simulink model "et_robocon_zack_stepup"  (R2013b)
settings: Solver=ode3  SolverMode=SingleTasking  StartTime=0.0  StopTime=inf  RelTol=1e-3
undefined symbols (not defined in the file): balancerStates_Bus0, current_mode_status, current_task_operation_status, DiscIntNeverNeededParam, Init_Bus0, K, lightCalib, R, STATE, TRACK_MODE_LIST, W
libraries: legonxtlib x19, simulink_extras x4, simulink x3, limbo_algorithm_atomic_sub_chart_library x1, line_tracking_algorithm_atomic_sub_chart_library x1, parking_algorithm_atomic_sub_chart_library x1
(part 1 of 2)
settings Model: DataDictionary=marioDict.sldd  ExtModeTrigDuration=2  Creator=mbiesiad  LastModifiedBy=jmodiset
settings ConfigSet: Description=Use this configuration to communicate between two robots. This robot is the master.
settings OptimizationCC: OptimizeModelRefInitCode=on  LifeSpan=1
settings DebuggingCC: UnderspecifiedInitializationDetection=Simplified  SolverPrmCheckMsg=none  ParameterPrecisionLossMsg=none  SignalLabelMismatchMsg=error  NonBusSignalsTreatedAsBus=error
settings HardwareCC: ProdLargestAtomicInteger=Long  ProdLargestAtomicFloat=Float  ProdEndianess=LittleEndian  ProdHWDeviceType=ARM Compatible->ARM 7
settings RTWCC: SystemTargetFile=realtime.tlc  GenerateMakefile=off  TemplateMakefile=realtime.tmf  Description=Run on Target Hardware  RTWVerbose=off  ProcessScript=realtime_make_rtw_hook
settings STFCustomTargetCC: TargetLibSuffix=.a  GenerateSampleERTMain=on  ERTCustomFileBanners=on  SupportNonInlinedSFcns=off  SupportVariableSizeSignals=on  MATLABClassNameForMDSCustomization=Simulink.SoftwareTarget.ERTCustomization  GRTInterface=off  SystemTargetFile=realtime.tlc
settings ERTTargetCC: CodeReplacementLibrary=ANSI_C  GenerateSampleERTMain=on  ParMdlRefBuildCompliant=off  CompOptLevelCompliant=off  ConcurrentExecutionCompliant=off  CombineOutputUpdateFcns=off  ERTFirstTimeCompliant=off  SupportContinuousTime=on  SupportVariableSizeSignals=on  ModelStepFunctionPrototypeControlCompliant=off  CPPClassGenCompliant=off  ExtModeTransport=1  ExtModeMexFile=ext_serial_win32_comm_no_acks_rtt_byteswap  ExtModeMexArgs=0 1 9600  InlinedParameterPlacement=NonHierarchical  ERTSrcFileBannerTemplate=realtime_code_template.cgt  ERTHdrFileBannerTemplate=realtime_code_template.cgt  ERTDataSrcFileTemplate=realtime_code_template.cgt  ERTDataHdrFileTemplate=realtime_code_template.cgt  ERTCustomFileTemplate=realtime_file_process.tlc

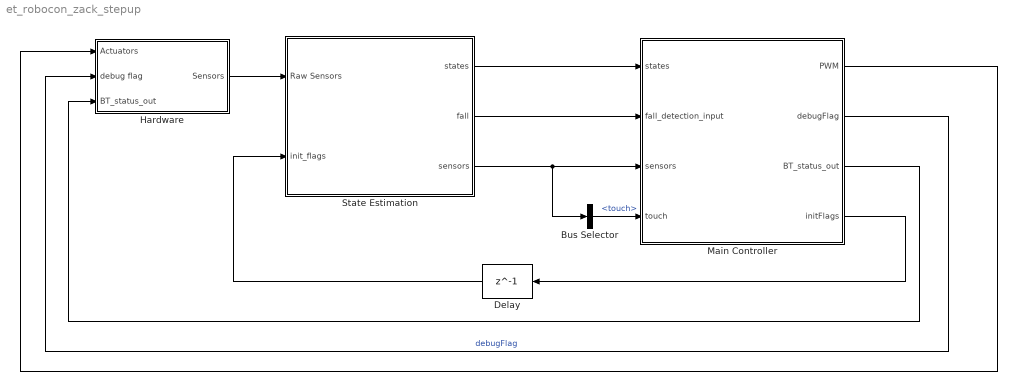
== system et_robocon_zack_stepup ==
  Bus Selector : BusSelector  OutputSignals=touch
  Delay : Delay  DelayLength=1
  Hardware : Subsystem  VariantControl=Variant1
  Main Controller : Stateflow chart  TreatAsAtomicUnit=on
  State Estimation : Subsystem
  wires:
  State Estimation/2(fall) -> Main Controller/2(fall_detection_input)
  State Estimation/3(sensors) -> Bus Selector/1, Main Controller/3(sensors)
  Bus Selector/1 -> Main Controller/4(touch)  "<touch>"
  Hardware/1(Sensors) -> State Estimation/1(Raw Sensors)
  Main Controller/4(initFlags) -> Delay/1
  State Estimation/1(states) -> Main Controller/1(states)
  Delay/1 -> State Estimation/2(init_flags)
  Main Controller/2(debugFlag) -> Hardware/2(debug flag)  "debugFlag"
  Main Controller/1(PWM) -> Hardware/1(Actuators)
  Main Controller/3(BT_status_out) -> Hardware/3(BT_status_out)

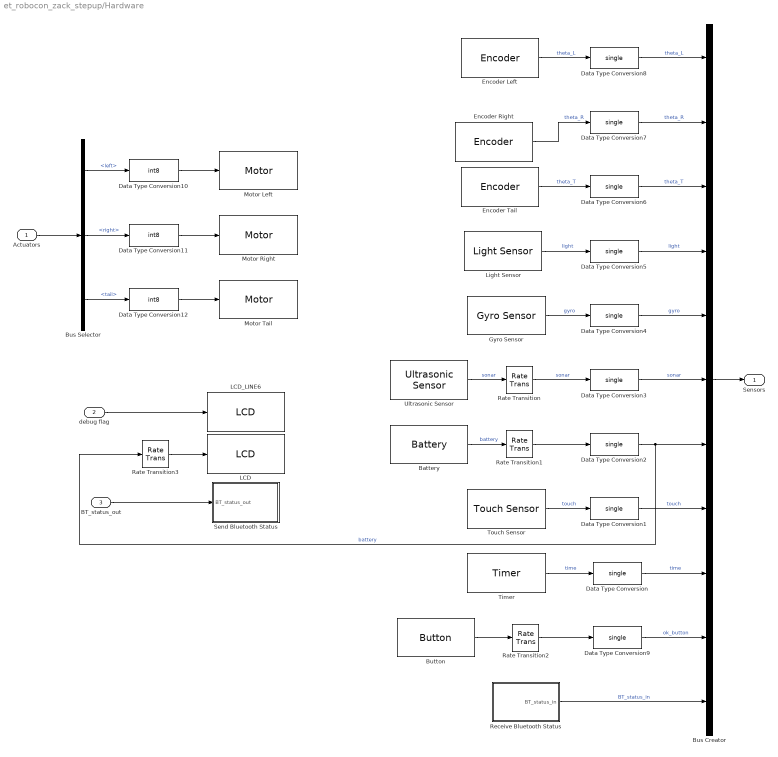
== system et_robocon_zack_stepup/Hardware ==
  Actuators : Inport
  debug flag : Inport  Port=2
  BT_status_out : Inport  Port=3
  Battery : legonxtlib/Battery  sampleTime=.1
  Bus Creator : BusCreator  Inputs=11
  Bus Selector : BusSelector  OutputSignals=left,right,tail
  Button : legonxtlib/Button  buttonType=Middle orange  sampleTime=0.1
  Data Type Conversion{,1..9} (10 alike) : DataTypeConversion  OutDataTypeStr=single
  Data Type Conversion10 : DataTypeConversion  OutDataTypeStr=int8  SaturateOnIntegerOverflow=on
  Data Type Conversion11 : DataTypeConversion  OutDataTypeStr=int8  SaturateOnIntegerOverflow=on
  Data Type Conversion12 : DataTypeConversion  OutDataTypeStr=int8  SaturateOnIntegerOverflow=on
  Encoder Left : legonxtlib/Encoder  portNumber=C  opMode=No reset  sampleTime=0.004
  Encoder Right : legonxtlib/Encoder  portNumber=B  opMode=No reset  sampleTime=0.004
  Encoder Tail : legonxtlib/Encoder  portNumber=A  opMode=No reset  sampleTime=0.004
  Gyro Sensor : legonxtlib/Gyro Sensor  portNumber=1  outputMode=Rotation rate (-360 - 360)  offset=600  sampleTime=0.004
  LCD : legonxtlib/LCD  slcdStr=Battery  slcdLine=2  slcdFormat=Decimal
  LCD_LINE6 : legonxtlib/LCD  slcdStr=STATE:  slcdLine=1  slcdFormat=Decimal
  Light Sensor : legonxtlib/Light Sensor  portNumber=3  outputMode=Raw A/D (1023 - 0)  lightOn=on  sampleTime=0.004
  Motor Left : legonxtlib/Motor  sportNumber=C  sstopAction=Brake
  Motor Right : legonxtlib/Motor  sportNumber=B  sstopAction=Brake
  Motor Tail : legonxtlib/Motor  sportNumber=A  sstopAction=Brake
  Rate Transition : RateTransition  OutPortSampleTime=0.004
  Rate Transition1 : RateTransition  OutPortSampleTime=0.004
  Rate Transition2 : RateTransition  OutPortSampleTime=0.004
  Rate Transition3 : RateTransition  OutPortSampleTime=3
  Receive Bluetooth Status : Subsystem  Variant=on
  Send Bluetooth Status : Subsystem  Variant=on
  Timer : legonxtlib/Timer  sampleTime=0.004
  Touch Sensor : legonxtlib/Touch Sensor  portNumber=4  sampleTime=0.004
  Ultrasonic Sensor : legonxtlib/Ultrasonic Sensor  PortNumber=2  sampleTime=0.02
  Sensors : Outport
  wires:
  Receive Bluetooth Status/1(BT_status_in) -> Bus Creator/11  "BT_status_in"
  debug flag/1 -> LCD_LINE6/1
  Data Type Conversion9/1 -> Bus Creator/10  "ok_button"
  Rate Transition2/1 -> Data Type Conversion9/1
  Button/1 -> Rate Transition2/1
  Rate Transition1/1 -> Data Type Conversion2/1
  Data Type Conversion8/1 -> Bus Creator/1  "theta_L"
  Data Type Conversion7/1 -> Bus Creator/2  "theta_R"
  Data Type Conversion6/1 -> Bus Creator/3  "theta_T"
  Data Type Conversion5/1 -> Bus Creator/4  "light"
  Data Type Conversion4/1 -> Bus Creator/5  "gyro"
  Data Type Conversion3/1 -> Bus Creator/6  "sonar"
  Data Type Conversion2/1 -> Rate Transition3/1, Bus Creator/7  "battery"
  Data Type Conversion1/1 -> Bus Creator/8  "touch"
  Data Type Conversion/1 -> Bus Creator/9  "time"
  Rate Transition/1 -> Data Type Conversion3/1  "sonar"
  Ultrasonic Sensor/1 -> Rate Transition/1  "sonar"
  Bus Selector/3 -> Data Type Conversion12/1  "<tail>"
  Encoder Tail/1 -> Data Type Conversion6/1  "theta_T"
  Light Sensor/1 -> Data Type Conversion5/1  "light"
  Bus Selector/2 -> Data Type Conversion11/1  "<right>"
  Bus Selector/1 -> Data Type Conversion10/1  "<left>"
  Touch Sensor/1 -> Data Type Conversion1/1  "touch"
  Bus Creator/1 -> Sensors/1
  Battery/1 -> Rate Transition1/1  "battery"
  Gyro Sensor/1 -> Data Type Conversion4/1  "gyro"
  Encoder Right/1 -> Data Type Conversion7/1  "theta_R"
  Encoder Left/1 -> Data Type Conversion8/1  "theta_L"
  Timer/1 -> Data Type Conversion/1  "time"
  Actuators/1 -> Bus Selector/1
  Data Type Conversion10/1 -> Motor Left/1
  Data Type Conversion11/1 -> Motor Right/1
  Data Type Conversion12/1 -> Motor Tail/1
  BT_status_out/1 -> Send Bluetooth Status/1(BT_status_out)
  Rate Transition3/1 -> LCD/1

== system et_robocon_zack_stepup/Main Controller/normal_operation_modes.gyro_calibration_mode ==
  sensors : Inport
  touch : Inport  Port=2
  " Demux " : Demux  Outputs=2
  " SFunction " : S-Function  Tag=Stateflow S-Function et_robocon_zack_stepup 5  FunctionName=sf_sfun  PortCounts=[3 6]  EnableBusSupport=off
  gyro_calibration_mode.GyroCalibration.Speak : Subsystem
      settings: UndoDeleteFcn=Stateflow.SLINSF.SimulinkMan.restorePreDeleteFcn  PreDeleteFcn=Stateflow.SLINSF.SimulinkMan.removePreDeleteFcn
  gyro_calibration_mode.GyroCalibration.tail_controller : Subsystem
      settings: UndoDeleteFcn=Stateflow.SLINSF.SimulinkMan.restorePreDeleteFcn  PreDeleteFcn=Stateflow.SLINSF.SimulinkMan.removePreDeleteFcn
  debugFlag : Outport
  initFlags : Outport  Port=2
  PWM : Outport  Port=3
  wires:
  sensors/1 -> " SFunction "/1
  touch/1 -> " SFunction "/2
  " SFunction "/2 -> debugFlag/1  "debugFlag"
  " SFunction "/3 -> initFlags/1  "initFlags"
  " SFunction "/4 -> PWM/1  "PWM"
  " SFunction "/5 -> gyro_calibration_mode.GyroCalibration.tail_controller/1(current)
  " SFunction "/6 -> gyro_calibration_mode.GyroCalibration.tail_controller/2(desired)
  gyro_calibration_mode.GyroCalibration.tail_controller/1(cmd) -> " SFunction "/3
  " Demux "/1 -> gyro_calibration_mode.GyroCalibration.tail_controller/Trigger
  " Demux "/2 -> gyro_calibration_mode.GyroCalibration.Speak/Trigger
  " SFunction "/1 -> " Demux "/1

== system et_robocon_zack_stepup/Main Controller/normal_operation_modes.light_sensor_calibration_mode ==
  sensors : Inport
  touch : Inport  Port=2
  " Demux " : Demux  Outputs=1
  " SFunction " : S-Function  Tag=Stateflow S-Function et_robocon_zack_stepup 6  FunctionName=sf_sfun  PortCounts=[3 5]  EnableBusSupport=off
  light_sensor_calibration_mode.tail_controller : Subsystem
      settings: UndoDeleteFcn=Stateflow.SLINSF.SimulinkMan.restorePreDeleteFcn  PreDeleteFcn=Stateflow.SLINSF.SimulinkMan.removePreDeleteFcn
  debugFlag : Outport
  PWM : Outport  Port=2
  wires:
  sensors/1 -> " SFunction "/1
  touch/1 -> " SFunction "/2
  " SFunction "/2 -> debugFlag/1  "debugFlag"
  " SFunction "/3 -> PWM/1  "PWM"
  " SFunction "/4 -> light_sensor_calibration_mode.tail_controller/1(current)
  " SFunction "/5 -> light_sensor_calibration_mode.tail_controller/2(desired)
  light_sensor_calibration_mode.tail_controller/1(cmd) -> " SFunction "/3
  " Demux "/1 -> light_sensor_calibration_mode.tail_controller/Trigger
  " SFunction "/1 -> " Demux "/1

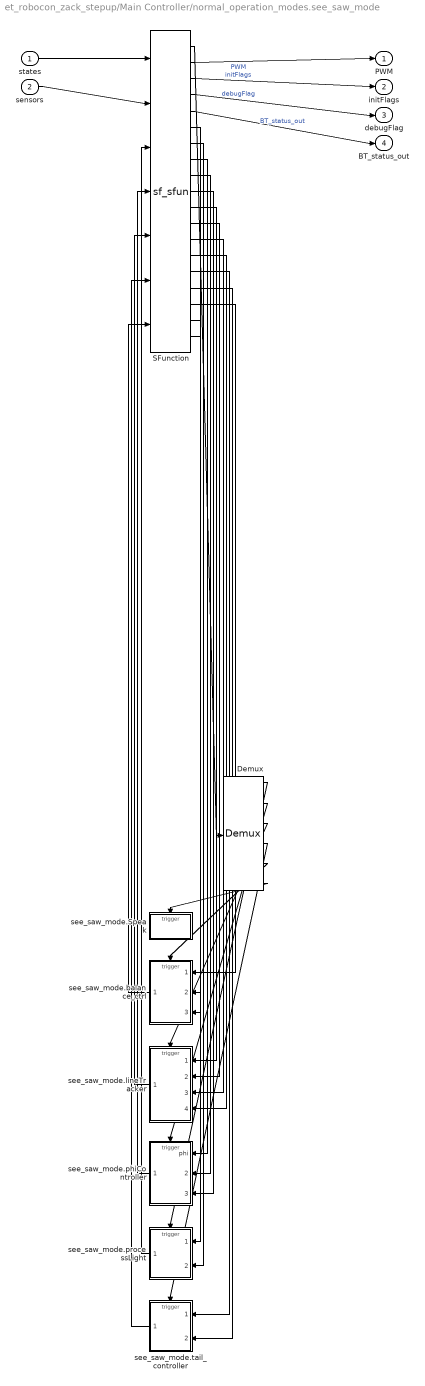
== system et_robocon_zack_stepup/Main Controller/normal_operation_modes.see_saw_mode ==
  states : Inport
  sensors : Inport  Port=2
  " Demux " : Demux  Outputs=6
  " SFunction " : S-Function  Tag=Stateflow S-Function et_robocon_zack_stepup 4  FunctionName=sf_sfun  Parameters=balancerStates_Bus0  PortCounts=[7 19]  EnableBusSupport=off
  see_saw_mode.Speak : Subsystem
      settings: UndoDeleteFcn=Stateflow.SLINSF.SimulinkMan.restorePreDeleteFcn  PreDeleteFcn=Stateflow.SLINSF.SimulinkMan.removePreDeleteFcn
  see_saw_mode.balance_ctrl : Subsystem
      settings: UndoDeleteFcn=Stateflow.SLINSF.SimulinkMan.restorePreDeleteFcn  PreDeleteFcn=Stateflow.SLINSF.SimulinkMan.removePreDeleteFcn
  see_saw_mode.lineTracker : Subsystem
      settings: UndoDeleteFcn=Stateflow.SLINSF.SimulinkMan.restorePreDeleteFcn  PreDeleteFcn=Stateflow.SLINSF.SimulinkMan.removePreDeleteFcn
  see_saw_mode.phiController : Subsystem
      settings: UndoDeleteFcn=Stateflow.SLINSF.SimulinkMan.restorePreDeleteFcn  PreDeleteFcn=Stateflow.SLINSF.SimulinkMan.removePreDeleteFcn
  see_saw_mode.processLight : Subsystem
      settings: UndoDeleteFcn=Stateflow.SLINSF.SimulinkMan.restorePreDeleteFcn  PreDeleteFcn=Stateflow.SLINSF.SimulinkMan.removePreDeleteFcn
  see_saw_mode.tail_controller : Subsystem
      settings: UndoDeleteFcn=Stateflow.SLINSF.SimulinkMan.restorePreDeleteFcn  PreDeleteFcn=Stateflow.SLINSF.SimulinkMan.removePreDeleteFcn
  PWM : Outport
  initFlags : Outport  Port=2
  debugFlag : Outport  Port=3
  BT_status_out : Outport  Port=4
  wires:
  states/1 -> " SFunction "/1
  sensors/1 -> " SFunction "/2
  " SFunction "/2 -> PWM/1  "PWM"
  " SFunction "/3 -> initFlags/1  "initFlags"
  " SFunction "/4 -> debugFlag/1  "debugFlag"
  " SFunction "/5 -> BT_status_out/1  "BT_status_out"
  " SFunction "/6 -> see_saw_mode.processLight/1(rawLight)
  " SFunction "/7 -> see_saw_mode.processLight/2(lightCalib)
  see_saw_mode.processLight/1(light) -> " SFunction "/3
  " Demux "/1 -> see_saw_mode.processLight/Trigger
  " SFunction "/8 -> see_saw_mode.phiController/1(phi)
  " SFunction "/9 -> see_saw_mode.phiController/2(desiredPhi)
  " SFunction "/10 -> see_saw_mode.phiController/3(battery)
  see_saw_mode.phiController/1(cmd) -> " SFunction "/4
  " Demux "/2 -> see_saw_mode.phiController/Trigger
  " SFunction "/11 -> see_saw_mode.lineTracker/1(desiredLight)
  " SFunction "/12 -> see_saw_mode.lineTracker/2(light)
  " SFunction "/13 -> see_saw_mode.lineTracker/3(trackingPower)
  " SFunction "/14 -> see_saw_mode.lineTracker/4(battery)
  see_saw_mode.lineTracker/1(cmd) -> " SFunction "/5
  " Demux "/3 -> see_saw_mode.lineTracker/Trigger
  " SFunction "/15 -> see_saw_mode.tail_controller/1(current)
  " SFunction "/16 -> see_saw_mode.tail_controller/2(desired)
  see_saw_mode.tail_controller/1(cmd) -> " SFunction "/6
  " Demux "/4 -> see_saw_mode.tail_controller/Trigger
  " SFunction "/17 -> see_saw_mode.balance_ctrl/1(balancerStates)
  " SFunction "/18 -> see_saw_mode.balance_ctrl/2(desired_velocity)
  " SFunction "/19 -> see_saw_mode.balance_ctrl/3(battery)
  see_saw_mode.balance_ctrl/1(cmd) -> " SFunction "/7
  " Demux "/5 -> see_saw_mode.balance_ctrl/Trigger
  " Demux "/6 -> see_saw_mode.Speak/Trigger
  " SFunction "/1 -> " Demux "/1

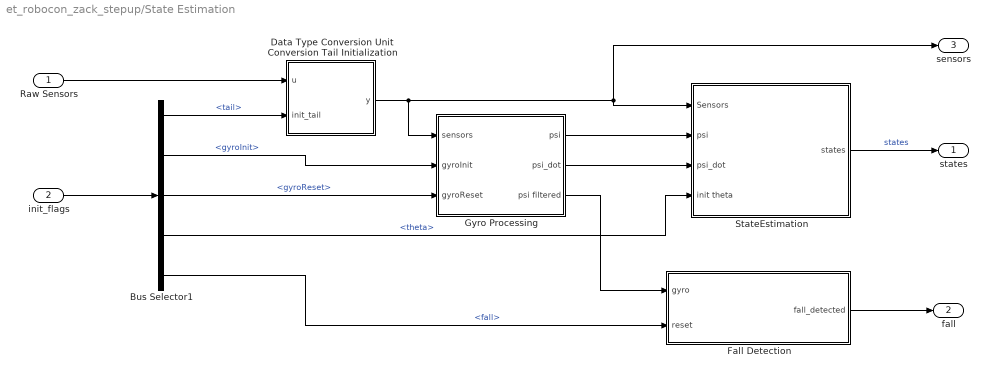
== system et_robocon_zack_stepup/State Estimation ==
  Raw Sensors : Inport
  init_flags : Inport  Port=2
  Bus Selector1 : BusSelector  OutputSignals=tail,gyroInit,gyroReset,theta,fall
  Data Type Conversion Unit Conversion Tail Initialization : Subsystem
  Fall Detection : Subsystem
  Gyro Processing : Subsystem
  StateEstimation : Subsystem
  states : Outport
  fall : Outport  Port=2
  sensors : Outport  Port=3
  wires:
  Bus Selector1/3 -> Gyro Processing/3(gyroReset)  "<gyroReset>"
  Bus Selector1/4 -> StateEstimation/4(init theta)  "<theta>"
  Bus Selector1/1 -> Data Type Conversion Unit Conversion Tail Initialization/2(init_tail)  "<tail>"
  Bus Selector1/2 -> Gyro Processing/2(gyroInit)  "<gyroInit>"
  init_flags/1 -> Bus Selector1/1
  StateEstimation/1(states) -> states/1  "states"
  Data Type Conversion Unit Conversion Tail Initialization/1(y) -> StateEstimation/1(Sensors), sensors/1, Gyro Processing/1(sensors)
  Raw Sensors/1 -> Data Type Conversion Unit Conversion Tail Initialization/1(u)
  Gyro Processing/1(psi) -> StateEstimation/2(psi)
  Gyro Processing/2(psi_dot) -> StateEstimation/3(psi_dot)
  Gyro Processing/3(psi filtered) -> Fall Detection/1(gyro)
  Bus Selector1/5 -> Fall Detection/2(reset)  "<fall>"
  Fall Detection/1(fall_detected) -> fall/1

== system et_robocon_zack_stepup/Hardware/Receive Bluetooth Status ==
  note: 1) Only subsystems can be added as variant choices at this level
      | 2) Blocks cannot be connected at this level as connectivity is
      | automatically determined at simulation, based on the active variant
  BluetoothOFF : Subsystem  VariantControl=BluetoothOFF
  BluetoothON : Subsystem  VariantControl=BluetoothON
  BT_status_in : Outport

== system et_robocon_zack_stepup/Hardware/Send Bluetooth Status ==
  note: 1) Only subsystems can be added as variant choices at this level
      | 2) Blocks cannot be connected at this level as connectivity is
      | automatically determined at simulation, based on the active variant
  BT_status_out : Inport
  BluetoothOFF : Subsystem  VariantControl=BluetoothOFF
  BluetoothON : Subsystem  VariantControl=BluetoothON

== system et_robocon_zack_stepup/Main Controller/normal_operation_modes.gyro_calibration_mode/gyro_calibration_mode.GyroCalibration.Speak ==
  f : TriggerPort  TriggerType=function-call
      settings: CopyFcn=Stateflow.SLINSF.SimulinkMan.removeBlockPreDeleteFcn  PreDeleteFcn=Stateflow.SLINSF.SimulinkMan.unsafePredeleteFcn
  Constant : Constant  Value=50
  Speaker : legonxtlib/Speaker  sinputMode=Volume only  sspeakerFreq=800  sspeakerVolume=50  sspeakerDuration=100
  wires:
  Constant/1 -> Speaker/1

== system et_robocon_zack_stepup/Main Controller/normal_operation_modes.gyro_calibration_mode/gyro_calibration_mode.GyroCalibration.tail_controller ==
  note: Could be improved, PI for example
  current : Inport  OutDataTypeStr=single  PortDimensions=1
  desired : Inport  Port=2  OutDataTypeStr=single  PortDimensions=1
  f : TriggerPort  TriggerType=function-call
      settings: CopyFcn=Stateflow.SLINSF.SimulinkMan.removeBlockPreDeleteFcn  PreDeleteFcn=Stateflow.SLINSF.SimulinkMan.unsafePredeleteFcn
  Gain : Gain  Gain=250
  Saturation : Saturate  UpperLimit=100  LowerLimit=-100  OutDataTypeStr=single
  Sum : Sum  Inputs=|+-
  cmd : Outport  OutDataTypeStr=single  PortDimensions=1  InitialOutput=0
  wires:
  Saturation/1 -> cmd/1
  Gain/1 -> Saturation/1
  desired/1 -> Sum/1
  current/1 -> Sum/2
  Sum/1 -> Gain/1

== system et_robocon_zack_stepup/Main Controller/normal_operation_modes.light_sensor_calibration_mode/light_sensor_calibration_mode.tail_controller ==
  note: Could be improved, PI for example
  current : Inport  OutDataTypeStr=single  PortDimensions=1
  desired : Inport  Port=2  OutDataTypeStr=single  PortDimensions=1
  f : TriggerPort  TriggerType=function-call
      settings: CopyFcn=Stateflow.SLINSF.SimulinkMan.removeBlockPreDeleteFcn  PreDeleteFcn=Stateflow.SLINSF.SimulinkMan.unsafePredeleteFcn
  Gain : Gain  Gain=250
  Saturation : Saturate  UpperLimit=100  LowerLimit=-100  OutDataTypeStr=single
  Sum : Sum  Inputs=|+-
  cmd : Outport  OutDataTypeStr=single  PortDimensions=1  InitialOutput=0
  wires:
  Saturation/1 -> cmd/1
  Gain/1 -> Saturation/1
  desired/1 -> Sum/1
  current/1 -> Sum/2
  Sum/1 -> Gain/1

== system et_robocon_zack_stepup/Main Controller/normal_operation_modes.see_saw_mode/see_saw_mode.Speak ==
  f : TriggerPort  TriggerType=function-call
      settings: CopyFcn=Stateflow.SLINSF.SimulinkMan.removeBlockPreDeleteFcn  PreDeleteFcn=Stateflow.SLINSF.SimulinkMan.unsafePredeleteFcn
  Constant : Constant  Value=50
  Speaker : legonxtlib/Speaker  sinputMode=Volume only  sspeakerFreq=800  sspeakerVolume=50  sspeakerDuration=100
  wires:
  Constant/1 -> Speaker/1

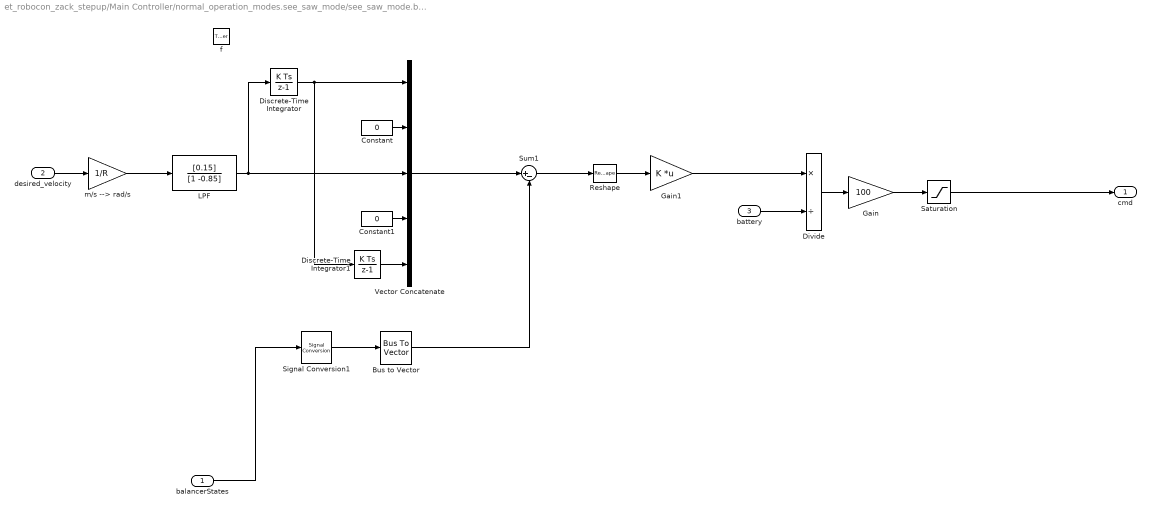
== system et_robocon_zack_stepup/Main Controller/normal_operation_modes.see_saw_mode/see_saw_mode.balance_ctrl ==
  balancerStates : Inport  OutDataTypeStr=Bus: Balancer_States_Bus  PortDimensions=1
  desired_velocity : Inport  Port=2  OutDataTypeStr=single  PortDimensions=1  BusOutputAsStruct=on
  battery : Inport  Port=3  OutDataTypeStr=double  PortDimensions=1
  f : TriggerPort  TriggerType=function-call
      settings: CopyFcn=Stateflow.SLINSF.SimulinkMan.removeBlockPreDeleteFcn  PreDeleteFcn=Stateflow.SLINSF.SimulinkMan.unsafePredeleteFcn
  Bus to Vector : BusToVector
  Constant : Constant  Value=0  OutDataTypeStr=single
  Constant1 : Constant  Value=0  OutDataTypeStr=single
  Discrete-Time Integrator : DiscreteIntegrator  SampleTime=-1  ICPrevOutput=DiscIntNeverNeededParam  ICPrevScaledInput=DiscIntNeverNeededParam
  Discrete-Time Integrator1 : DiscreteIntegrator  SampleTime=-1  ICPrevOutput=DiscIntNeverNeededParam  ICPrevScaledInput=DiscIntNeverNeededParam
  Divide : Product  Inputs=*/
  Gain : Gain  Gain=100
  Gain1 : Gain  Gain=K  Multiplication=Matrix(K*u)
  LPF : DiscreteFilter  Numerator=[0.15]  Denominator=[1 -0.85]
  Reshape : Reshape  OutputDimensionality=Column vector (2-D)
  Saturation : Saturate  UpperLimit=100  LowerLimit=-100  OutDataTypeStr=single
  Signal Conversion1 : SignalConversion  ConversionOutput=Virtual bus
  Sum1 : Sum  Inputs=|+-
  Vector Concatenate : Concatenate  NumInputs=5
  m/s --> rad/s : Gain  Gain=1/R
  cmd : Outport  OutDataTypeStr=single  PortDimensions=1  InitialOutput=0
  wires:
  Discrete-Time Integrator1/1 -> Vector Concatenate/5
  Discrete-Time Integrator/1 -> Vector Concatenate/1, Discrete-Time Integrator1/1
  Constant1/1 -> Vector Concatenate/4
  LPF/1 -> Vector Concatenate/3, Discrete-Time Integrator/1
  Constant/1 -> Vector Concatenate/2
  m/s --> rad/s/1 -> LPF/1
  Signal Conversion1/1 -> Bus to Vector/1
  Divide/1 -> Gain/1
  Gain/1 -> Saturation/1
  Gain1/1 -> Divide/1
  Saturation/1 -> cmd/1
  battery/1 -> Divide/2
  Vector Concatenate/1 -> Sum1/1
  balancerStates/1 -> Signal Conversion1/1
  Bus to Vector/1 -> Sum1/2
  desired_velocity/1 -> m/s --> rad/s/1
  Sum1/1 -> Reshape/1
  Reshape/1 -> Gain1/1

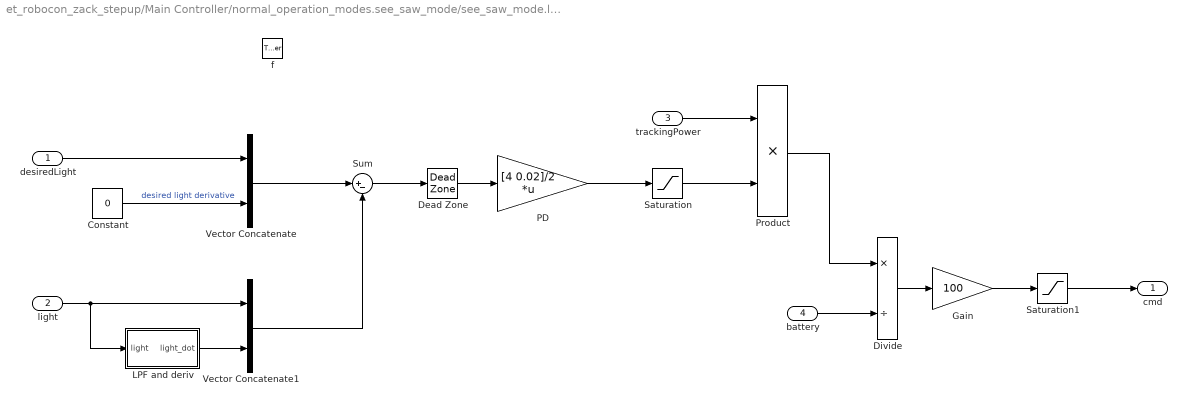
== system et_robocon_zack_stepup/Main Controller/normal_operation_modes.see_saw_mode/see_saw_mode.lineTracker ==
  desiredLight : Inport  OutDataTypeStr=single  PortDimensions=1
  light : Inport  Port=2  OutDataTypeStr=single  PortDimensions=1
  trackingPower : Inport  Port=3  OutDataTypeStr=single  PortDimensions=1
  battery : Inport  Port=4  OutDataTypeStr=double  PortDimensions=1
  f : TriggerPort  TriggerType=function-call
      settings: CopyFcn=Stateflow.SLINSF.SimulinkMan.removeBlockPreDeleteFcn  PreDeleteFcn=Stateflow.SLINSF.SimulinkMan.unsafePredeleteFcn
  Constant : Constant  Value=0  OutDataTypeStr=single
  Dead Zone : DeadZone  LowerValue=-0.02  UpperValue=0.02  SaturateOnIntegerOverflow=on
  Divide : Product  Inputs=*/
  Gain : Gain  Gain=100
  LPF and deriv : Subsystem
  PD : Gain  Gain="[4  0.02]/2"  Multiplication=Matrix(K*u)
  Product : Product
  Saturation : Saturate  UpperLimit=6  LowerLimit=-6
  Saturation1 : Saturate  UpperLimit=100  LowerLimit=-100  OutDataTypeStr=single
  Sum : Sum  Inputs=|+-
  Vector Concatenate : Concatenate
  Vector Concatenate1 : Concatenate
  cmd : Outport  OutDataTypeStr=single  PortDimensions=1
  wires:
  Divide/1 -> Gain/1
  Gain/1 -> Saturation1/1
  battery/1 -> Divide/2
  Saturation1/1 -> cmd/1
  Product/1 -> Divide/1
  trackingPower/1 -> Product/1
  Saturation/1 -> Product/2
  PD/1 -> Saturation/1
  Dead Zone/1 -> PD/1
  Sum/1 -> Dead Zone/1
  Vector Concatenate1/1 -> Sum/2
  Vector Concatenate/1 -> Sum/1
  light/1 -> Vector Concatenate1/1, LPF and deriv/1(light)
  LPF and deriv/1(light_dot) -> Vector Concatenate1/2
  Constant/1 -> Vector Concatenate/2  "desired light derivative"
  desiredLight/1 -> Vector Concatenate/1

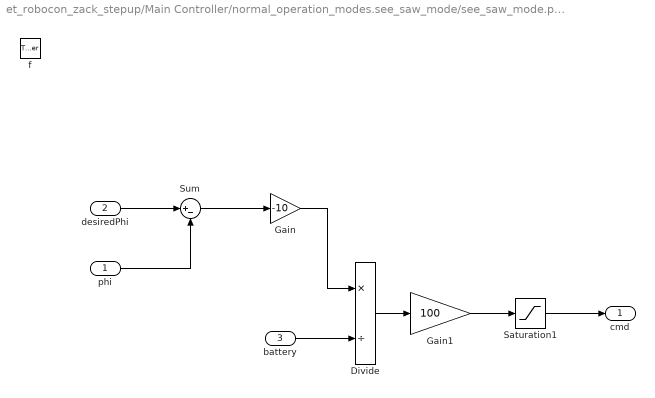
== system et_robocon_zack_stepup/Main Controller/normal_operation_modes.see_saw_mode/see_saw_mode.phiController ==
  phi : Inport  OutDataTypeStr=single  PortDimensions=1
  desiredPhi : Inport  Port=2  OutDataTypeStr=single  PortDimensions=1
  battery : Inport  Port=3  OutDataTypeStr=double  PortDimensions=1
  f : TriggerPort  TriggerType=function-call
      settings: CopyFcn=Stateflow.SLINSF.SimulinkMan.removeBlockPreDeleteFcn  PreDeleteFcn=Stateflow.SLINSF.SimulinkMan.unsafePredeleteFcn
  Divide : Product  Inputs=*/
  Gain : Gain  Gain=-10
  Gain1 : Gain  Gain=100
  Saturation1 : Saturate  UpperLimit=100  LowerLimit=-100  OutDataTypeStr=single
  Sum : Sum  Inputs=|+-
  cmd : Outport
  wires:
  Saturation1/1 -> cmd/1
  Gain/1 -> Divide/1
  Divide/1 -> Gain1/1
  Gain1/1 -> Saturation1/1
  battery/1 -> Divide/2
  Sum/1 -> Gain/1
  phi/1 -> Sum/2
  desiredPhi/1 -> Sum/1

== system et_robocon_zack_stepup/Main Controller/normal_operation_modes.see_saw_mode/see_saw_mode.processLight ==
  rawLight : Inport  OutDataTypeStr=single  PortDimensions=1
  lightCalib : Inport  Port=2  OutDataTypeStr=Bus: Light_Bus  PortDimensions=1
  f : TriggerPort  TriggerType=function-call
      settings: CopyFcn=Stateflow.SLINSF.SimulinkMan.removeBlockPreDeleteFcn  PreDeleteFcn=Stateflow.SLINSF.SimulinkMan.unsafePredeleteFcn
  Bus Selector : BusSelector  OutputSignals=black,white
  Gain : Gain  Gain=0.3
  Gain1 : Gain  Gain=1/100
  Sum : Sum  Inputs=|+-
  Sum1 : Sum  Inputs=|++
  Sum2 : Sum  Inputs=|+-
  light : Outport
  wires:
  Gain1/1 -> light/1
  Sum2/1 -> Gain1/1
  Sum1/1 -> Sum2/2
  rawLight/1 -> Sum2/1
  Gain/1 -> Sum1/1
  Sum/1 -> Gain/1
  Bus Selector/2 -> Sum/2, Sum1/2  "<white>"
  Bus Selector/1 -> Sum/1  "<black>"
  lightCalib/1 -> Bus Selector/1

== system et_robocon_zack_stepup/Main Controller/normal_operation_modes.see_saw_mode/see_saw_mode.tail_controller ==
  note: Could be improved, PI for example
  current : Inport  OutDataTypeStr=single  PortDimensions=1
  desired : Inport  Port=2  OutDataTypeStr=single  PortDimensions=1
  f : TriggerPort  TriggerType=function-call
      settings: CopyFcn=Stateflow.SLINSF.SimulinkMan.removeBlockPreDeleteFcn  PreDeleteFcn=Stateflow.SLINSF.SimulinkMan.unsafePredeleteFcn
  Gain : Gain  Gain=250
  Saturation : Saturate  UpperLimit=100  LowerLimit=-100  OutDataTypeStr=single
  Sum : Sum  Inputs=|+-
  cmd : Outport  OutDataTypeStr=single  PortDimensions=1  InitialOutput=0
  wires:
  Saturation/1 -> cmd/1
  Gain/1 -> Saturation/1
  desired/1 -> Sum/1
  current/1 -> Sum/2
  Sum/1 -> Gain/1

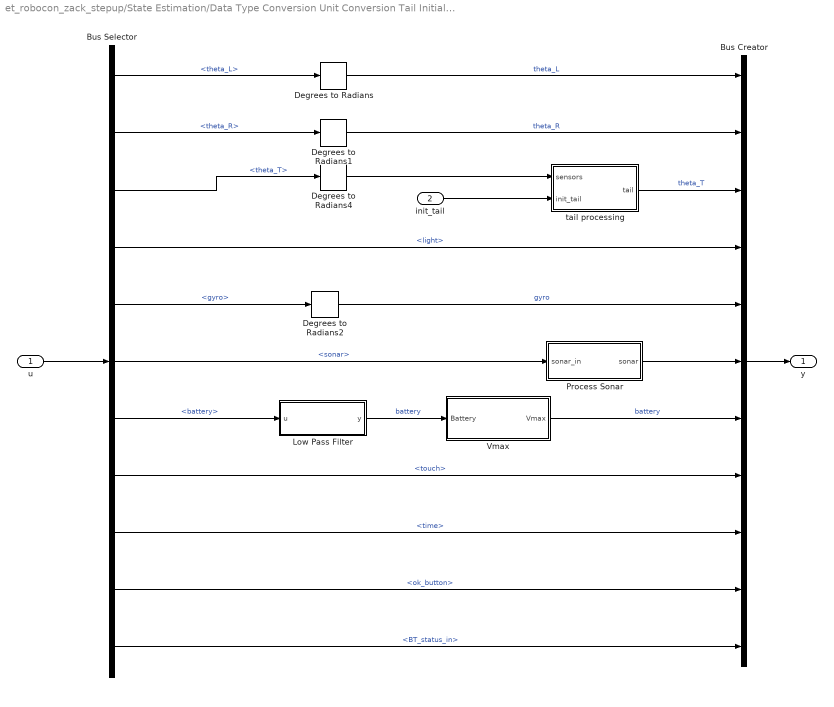
== system et_robocon_zack_stepup/State Estimation/Data Type Conversion Unit Conversion Tail Initialization ==
  u : Inport
  init_tail : Inport  Port=2
  Bus Creator : BusCreator  Inputs=11  OutDataTypeStr=Bus: Sensors_Bus
  Bus Selector : BusSelector  OutputSignals=theta_L,theta_R,theta_T,light,gyro,sonar,battery,touch,time,ok_button,BT_status_in
  Degrees to Radians{,1..2,4} (4 alike) : simulink_extras/Transformations/Degrees to Radians
  Low Pass Filter : Subsystem
  Process Sonar : Subsystem
  Vmax : Subsystem
  tail processing : Subsystem
  y : Outport
  wires:
  Bus Selector/11 -> Bus Creator/11  "<BT_status_in>"
  Process Sonar/1(sonar) -> Bus Creator/6
  Bus Selector/6 -> Process Sonar/1(sonar_in)  "<sonar>"
  Bus Selector/10 -> Bus Creator/10  "<ok_button>"
  init_tail/1 -> tail processing/2(init_tail)
  Bus Selector/9 -> Bus Creator/9  "<time>"
  Bus Selector/8 -> Bus Creator/8  "<touch>"
  tail processing/1(tail) -> Bus Creator/3  "theta_T"
  Degrees to Radians4/1 -> tail processing/1(sensors)
  Vmax/1(Vmax) -> Bus Creator/7  "battery"
  Degrees to Radians2/1 -> Bus Creator/5  "gyro"
  Bus Selector/3 -> Degrees to Radians4/1  "<theta_T>"
  Bus Selector/7 -> Low Pass Filter/1(u)  "<battery>"
  Bus Selector/5 -> Degrees to Radians2/1  "<gyro>"
  Bus Selector/4 -> Bus Creator/4  "<light>"
  Bus Creator/1 -> y/1
  u/1 -> Bus Selector/1
  Degrees to Radians/1 -> Bus Creator/1  "theta_L"
  Bus Selector/2 -> Degrees to Radians1/1  "<theta_R>"
  Bus Selector/1 -> Degrees to Radians/1  "<theta_L>"
  Low Pass Filter/1(y) -> Vmax/1(Battery)  "battery"
  Degrees to Radians1/1 -> Bus Creator/2  "theta_R"

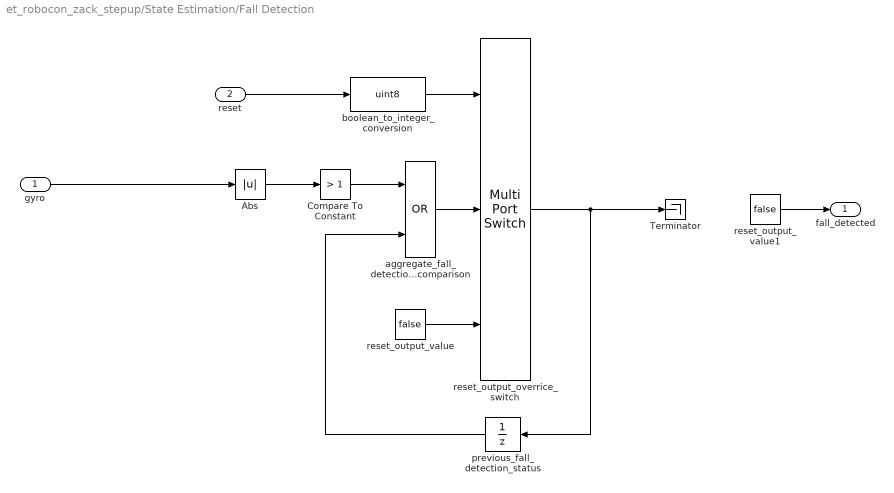
== system et_robocon_zack_stepup/State Estimation/Fall Detection ==
  gyro : Inport
      settings: AttributesFormatString=Output data type: %<OutDataTypeStr>
  reset : Inport  Port=2  OutDataTypeStr=boolean
      settings: AttributesFormatString=Output data type: %<OutDataTypeStr>
  Abs : Abs
  Compare To Constant : simulink/Logic and Bit Operations/Compare To Constant  relop=>  const=1  OutDataTypeStr=boolean
  Terminator : Terminator
  aggregate_fall_detection_comparison : Logic  Operator=OR  OutDataTypeStr=boolean
  boolean_to_integer_conversion : DataTypeConversion  OutDataTypeStr=uint8
      settings: AttributesFormatString=Output data type: %<OutDataTypeStr>
  previous_fall_detection_status : UnitDelay  SampleTime=-1
  reset_output_overrice_switch : MultiPortSwitch  DataPortOrder=Zero-based contiguous  Inputs=2  zeroidx=on  InputSameDT=on
  reset_output_value : Constant  Value=false
  reset_output_value1 : Constant  Value=false
  fall_detected : Outport
  wires:
  reset_output_overrice_switch/1 -> Terminator/1, previous_fall_detection_status/1
  reset_output_value/1 -> reset_output_overrice_switch/3
  aggregate_fall_detection_comparison/1 -> reset_output_overrice_switch/2
  boolean_to_integer_conversion/1 -> reset_output_overrice_switch/1
  reset/1 -> boolean_to_integer_conversion/1
  previous_fall_detection_status/1 -> aggregate_fall_detection_comparison/2
  Abs/1 -> Compare To Constant/1
  gyro/1 -> Abs/1
  Compare To Constant/1 -> aggregate_fall_detection_comparison/1
  reset_output_value1/1 -> fall_detected/1

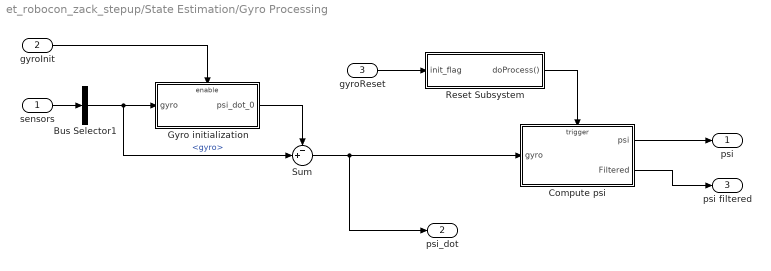
== system et_robocon_zack_stepup/State Estimation/Gyro Processing ==
  sensors : Inport
  gyroInit : Inport  Port=2
  gyroReset : Inport  Port=3
  Bus Selector1 : BusSelector  OutputSignals=gyro
  Compute psi : Subsystem
  Gyro initialization : Subsystem  TreatAsAtomicUnit=on
  Reset Subsystem : Stateflow chart  TreatAsAtomicUnit=on
  Sum : Sum  Inputs=-+|
  psi : Outport
  psi_dot : Outport  Port=2
  psi filtered : Outport  Port=3
  wires:
  Compute psi/2(Filtered) -> psi filtered/1
  Reset Subsystem/1(doProcess()) -> Compute psi/Trigger
  gyroReset/1 -> Reset Subsystem/1(init_flag)
  Bus Selector1/1 -> Sum/2, Gyro initialization/1(gyro)  "<gyro>"
  Gyro initialization/1(psi_dot_0) -> Sum/1
  Sum/1 -> psi_dot/1, Compute psi/1(gyro)
  Compute psi/1(psi) -> psi/1
  sensors/1 -> Bus Selector1/1
  gyroInit/1 -> Gyro initialization/Enable

== system et_robocon_zack_stepup/State Estimation/StateEstimation ==
  note: Conversion from Raw Sensors to States as described in "NXTway plant model.pdf"
  Sensors : Inport
  psi : Inport  Port=2
  psi_dot : Inport  Port=3
  init theta : Inport  Port=4
  Bus Creator1 : BusCreator  OutDataTypeStr=Bus: States_Bus
  Bus Creator2 : BusCreator  Inputs=5  OutDataTypeStr=Bus: Balancer_States_Bus
  Bus Selector1 : BusSelector  OutputSignals=theta_L,theta_R
  Process theta1 : Subsystem
  Reset Subsystem : Stateflow chart  TreatAsAtomicUnit=on
  states : Outport  OutputWhenDisabled=reset  InitialOutput=0
  wires:
  Process theta1/2(psi_out) -> Bus Creator2/2  "psi"
  Reset Subsystem/1(doProcess()) -> Process theta1/Trigger
  Bus Selector1/2 -> Process theta1/3(theta_r)  "<theta_R>"
  Bus Selector1/1 -> Process theta1/2(theta_l)  "<theta_L>"
  init theta/1 -> Reset Subsystem/1(init_flag)
  Process theta1/1(theta) -> Bus Creator2/1  "theta"
  Process theta1/3(theta_dot) -> Bus Creator2/3
  Process theta1/4(int_theta) -> Bus Creator2/5
  psi_dot/1 -> Bus Creator2/4  "psi_dot"
  Process theta1/6(phi_dot) -> Bus Creator1/3  "phi_dot"
  Bus Creator2/1 -> Bus Creator1/1  "balancerStates"
  Process theta1/5(phi) -> Bus Creator1/2  "phi"
  Sensors/1 -> Bus Selector1/1
  psi/1 -> Process theta1/1(psi)
  Bus Creator1/1 -> states/1
  Process theta1/7(theta_dot_dot) -> Bus Creator1/4  "theta_dot_dot"

== system et_robocon_zack_stepup/Hardware/Receive Bluetooth Status/BluetoothOFF ==
  Constant : Constant  Value=single(0)
  BT_status_in : Outport
  wires:
  Constant/1 -> BT_status_in/1

== system et_robocon_zack_stepup/Hardware/Receive Bluetooth Status/BluetoothON ==
  Data Type Conversion9 : DataTypeConversion  OutDataTypeStr=single
  Rate Transition2 : RateTransition  OutPortSampleTime=0.004
  Receive via Bluetooth(R) Connection : legonxtlib/Receive via Bluetooth(R) Connection  mailbox=1  dataType=uint8  dataSize=1  sampleTime=0.1
  BT_status_in : Outport
  wires:
  Data Type Conversion9/1 -> BT_status_in/1
  Rate Transition2/1 -> Data Type Conversion9/1
  Receive via Bluetooth(R) Connection/1 -> Rate Transition2/1

== system et_robocon_zack_stepup/Hardware/Send Bluetooth Status/BluetoothOFF ==
  BT_status_out : Inport
  Terminator : Terminator
  wires:
  BT_status_out/1 -> Terminator/1

== system et_robocon_zack_stepup/Hardware/Send Bluetooth Status/BluetoothON ==
  BT_status_out : Inport
  Data Type Conversion1 : DataTypeConversion  OutDataTypeStr=uint8
  Rate Transition1 : RateTransition  OutPortSampleTime=0.1
  Send via Bluetooth(R) Connection : legonxtlib/Send via Bluetooth(R) Connection  mailbox=2
  wires:
  BT_status_out/1 -> Rate Transition1/1
  Rate Transition1/1 -> Data Type Conversion1/1
  Data Type Conversion1/1 -> Send via Bluetooth(R) Connection/1

== system et_robocon_zack_stepup/Main Controller/normal_operation_modes.see_saw_mode/see_saw_mode.lineTracker/LPF and deriv ==
  light : Inport
  Discrete Filter : DiscreteFilter  Numerator=[0.05]  Denominator=[1 -0.95]
  Gain : Gain  Gain=1/0.004
  Sum3 : Sum  Inputs=+-
  Unit Delay : UnitDelay  SampleTime=-1
  light_dot : Outport
  wires:
  Unit Delay/1 -> Sum3/2
  Gain/1 -> Unit Delay/1, Sum3/1
  Sum3/1 -> light_dot/1  "theta_dot_dot"
  Discrete Filter/1 -> Gain/1
  light/1 -> Discrete Filter/1

== system et_robocon_zack_stepup/State Estimation/Data Type Conversion Unit Conversion Tail Initialization/Low Pass Filter ==
  u : Inport
  Constant : Constant  Value=0  OutDataTypeStr=boolean
  Low Pass Filter : DiscreteFilter  Numerator=[.01]  Denominator=[1 -0.99]
  Memory : Memory  X0=1  InheritSampleTime=on
  Store Offset : Subsystem  TreatAsAtomicUnit=on
  Sum1 : Sum  Inputs=++|
  Sum2 : Sum  Inputs=-+|
  y : Outport
  wires:
  Store Offset/1(x0) -> Sum1/1, Sum2/1
  u/1 -> Store Offset/1(x), Sum2/2
  Constant/1 -> Memory/1
  Memory/1 -> Store Offset/Enable
  Sum2/1 -> Low Pass Filter/1
  Sum1/1 -> y/1
  Low Pass Filter/1 -> Sum1/2

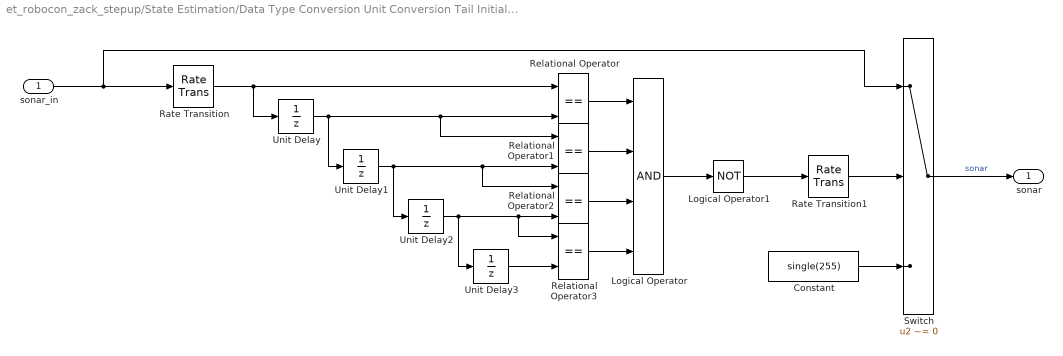
== system et_robocon_zack_stepup/State Estimation/Data Type Conversion Unit Conversion Tail Initialization/Process Sonar ==
  sonar_in : Inport
  Constant : Constant  Value=single(255)
  Logical Operator : Logic  Inputs=4  AllPortsSameDT=off  OutDataTypeStr=boolean
  Logical Operator1 : Logic  Operator=NOT  AllPortsSameDT=off  OutDataTypeStr=boolean
  Rate Transition : RateTransition  OutPortSampleTime=0.02
  Rate Transition1 : RateTransition  OutPortSampleTime=0.004
  Relational Operator{,1..3} (4 alike) : RelationalOperator  Operator===  OutDataTypeStr=boolean
  Switch : Switch  Criteria=u2 ~= 0
  Unit Delay{,1..3} (4 alike) : UnitDelay  SampleTime=-1
  sonar : Outport
  wires:
  Switch/1 -> sonar/1  "sonar"
  Constant/1 -> Switch/3
  Rate Transition1/1 -> Switch/2
  Logical Operator1/1 -> Rate Transition1/1
  Logical Operator/1 -> Logical Operator1/1
  Relational Operator2/1 -> Logical Operator/3
  Relational Operator1/1 -> Logical Operator/2
  Relational Operator3/1 -> Logical Operator/4
  Relational Operator/1 -> Logical Operator/1
  Unit Delay3/1 -> Relational Operator3/2
  Unit Delay2/1 -> Unit Delay3/1, Relational Operator2/2, Relational Operator3/1
  Unit Delay1/1 -> Unit Delay2/1, Relational Operator1/2, Relational Operator2/1
  Unit Delay/1 -> Unit Delay1/1, Relational Operator/2, Relational Operator1/1
  Rate Transition/1 -> Unit Delay/1, Relational Operator/1
  sonar_in/1 -> Rate Transition/1, Switch/1

== system et_robocon_zack_stepup/State Estimation/Data Type Conversion Unit Conversion Tail Initialization/Vmax ==
  Battery : Inport
  Constant : Constant  Value=0.625  OutDataTypeStr=single
  Gain1 : Gain  Gain=0.001089
  Sum : Sum  Inputs=|+-
  Vmax : Outport
  wires:
  Battery/1 -> Gain1/1
  Gain1/1 -> Sum/1
  Constant/1 -> Sum/2
  Sum/1 -> Vmax/1

== system et_robocon_zack_stepup/State Estimation/Data Type Conversion Unit Conversion Tail Initialization/tail processing ==
  sensors : Inport
  init_tail : Inport  Port=2
  Sum : Sum  Inputs=-+|
  tail initialization : Subsystem  TreatAsAtomicUnit=on
  tail : Outport  OutputWhenDisabled=reset  InitialOutput=0
  wires:
  Sum/1 -> tail/1  "theta_T"
  sensors/1 -> Sum/2, tail initialization/1(tail)
  tail initialization/1(tail_0) -> Sum/1
  init_tail/1 -> tail initialization/Trigger

== system et_robocon_zack_stepup/State Estimation/Gyro Processing/Compute psi ==
  gyro : Inport
  Trigger : TriggerPort  TriggerType=function-call  StatesWhenEnabling=reset  PortDimensions=1
  Discrete-Time Integrator : DiscreteIntegrator  SampleTime=-1  ICPrevOutput=DiscIntNeverNeededParam  ICPrevScaledInput=DiscIntNeverNeededParam
  Discrete-Time Integrator1 : DiscreteIntegrator  SampleTime=-1  ICPrevOutput=DiscIntNeverNeededParam  ICPrevScaledInput=DiscIntNeverNeededParam
  Sum3 : Sum  Inputs=|+-
  Very Low Pass Filter : Subsystem
  psi : Outport  InitialOutput=0
  Filtered : Outport  Port=2  InitialOutput=0
  wires:
  Discrete-Time Integrator/1 -> Filtered/1
  Discrete-Time Integrator1/1 -> psi/1
  Sum3/1 -> Discrete-Time Integrator/1
  Very Low Pass Filter/1(Out1) -> Sum3/2
  gyro/1 -> Very Low Pass Filter/1(In1), Sum3/1, Discrete-Time Integrator1/1

== system et_robocon_zack_stepup/State Estimation/Gyro Processing/Gyro initialization ==
  gyro : Inport
  Enable : EnablePort  StatesWhenEnabling=reset
  Low Pass Filter : DiscreteFilter  Numerator=[.01]  Denominator=[1 -0.99]
  psi_dot_0 : Outport  InitialOutput=0
  wires:
  Low Pass Filter/1 -> psi_dot_0/1
  gyro/1 -> Low Pass Filter/1

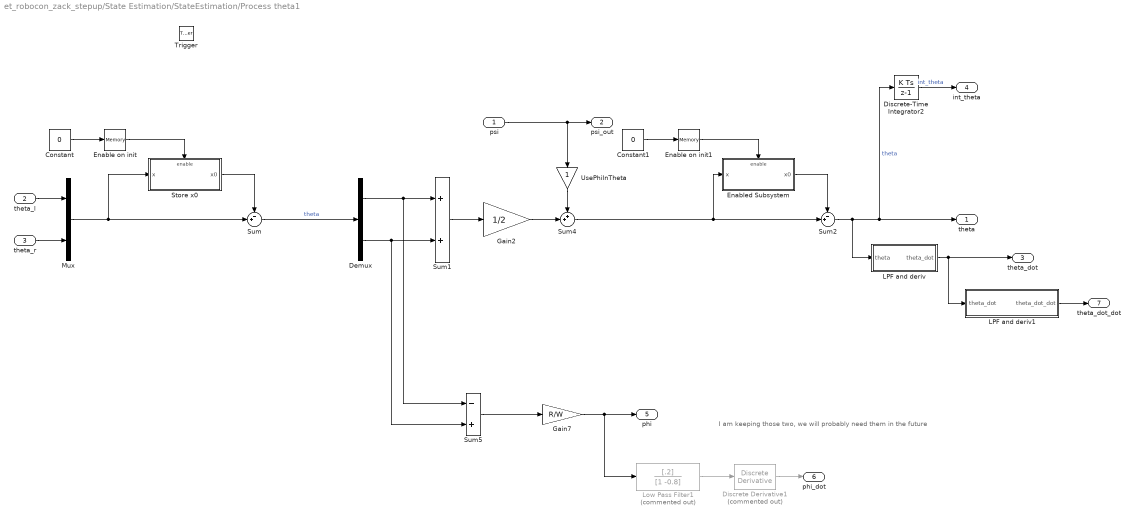
== system et_robocon_zack_stepup/State Estimation/StateEstimation/Process theta1 ==
  note: I am keeping those two, we will probably need them in the future
  psi : Inport
  theta_l : Inport  Port=2
  theta_r : Inport  Port=3
  Trigger : TriggerPort  TriggerType=function-call  StatesWhenEnabling=reset  PortDimensions=1
  Constant : Constant  Value=0  OutDataTypeStr=boolean
  Constant1 : Constant  Value=0  OutDataTypeStr=boolean
  Demux : Demux  Outputs=2
  Discrete Derivative1 : simulink/Discrete/Discrete Derivative  Commented=on  gainval=1.0  ICPrevScaledInput=0.0  InputProcessing=Inherited  OutMin=[]  OutMax=[]  OutDataType=fixdt(1, 16)  OutScaling=2^-10  DoSatur=off
  Discrete-Time Integrator2 : DiscreteIntegrator  SampleTime=-1  ICPrevOutput=DiscIntNeverNeededParam  ICPrevScaledInput=DiscIntNeverNeededParam
  Enable on init : Memory  X0=1  InheritSampleTime=on
  Enable on init1 : Memory  X0=1  InheritSampleTime=on
  Enabled Subsystem : Subsystem  TreatAsAtomicUnit=on
  Gain2 : Gain  Gain=1/2
  Gain7 : Gain  Gain=R/W
  LPF and deriv : Subsystem
  LPF and deriv1 : Subsystem
  Low Pass Filter1 : DiscreteFilter  Commented=on  Numerator=[.2]  Denominator=[1 -0.8]
  Mux : Mux  Inputs=2
  Store x0 : Subsystem  TreatAsAtomicUnit=on
  Sum : Sum  Inputs=-+|
  Sum1 : Sum
  Sum2 : Sum  Inputs=-+|
  Sum4 : Sum  Inputs=++|
  Sum5 : Sum  Inputs=-+
  UsePhiInTheta : Gain
  theta : Outport  InitialOutput=0
  psi_out : Outport  Port=2  InitialOutput=0
  theta_dot : Outport  Port=3  OutputWhenDisabled=reset  InitialOutput=0
  int_theta : Outport  Port=4  InitialOutput=0
  phi : Outport  Port=5  OutputWhenDisabled=reset  InitialOutput=0
  phi_dot : Outport  Port=6  OutputWhenDisabled=reset  InitialOutput=0
  theta_dot_dot : Outport  Port=7  OutputWhenDisabled=reset  InitialOutput=0
  wires:
  Gain7/1 -> Low Pass Filter1/1, phi/1
  Sum5/1 -> Gain7/1
  Sum2/1 -> LPF and deriv/1(theta), theta/1, Discrete-Time Integrator2/1  "theta"
  Enabled Subsystem/1(x0) -> Sum2/1
  Constant1/1 -> Enable on init1/1
  Enable on init1/1 -> Enabled Subsystem/Enable
  Sum4/1 -> Sum2/2, Enabled Subsystem/1(x)
  Discrete-Time Integrator2/1 -> int_theta/1  "int_theta"
  psi/1 -> UsePhiInTheta/1, psi_out/1
  UsePhiInTheta/1 -> Sum4/1
  Sum1/1 -> Gain2/1
  Gain2/1 -> Sum4/2
  Demux/2 -> Sum1/2, Sum5/2
  Demux/1 -> Sum1/1, Sum5/1
  theta_r/1 -> Mux/2
  theta_l/1 -> Mux/1
  Mux/1 -> Sum/2, Store x0/1(x)
  Sum/1 -> Demux/1  "theta"
  Store x0/1(x0) -> Sum/1
  Constant/1 -> Enable on init/1
  Enable on init/1 -> Store x0/Enable
  Low Pass Filter1/1 -> Discrete Derivative1/1
  Discrete Derivative1/1 -> phi_dot/1
  LPF and deriv/1(theta_dot) -> LPF and deriv1/1(theta_dot), theta_dot/1
  LPF and deriv1/1(theta_dot_dot) -> theta_dot_dot/1

== system et_robocon_zack_stepup/State Estimation/Data Type Conversion Unit Conversion Tail Initialization/Low Pass Filter/Store Offset ==
  x : Inport
  Enable : EnablePort
  x0 : Outport  InitialOutput=0
  wires:
  x/1 -> x0/1

== system et_robocon_zack_stepup/State Estimation/Data Type Conversion Unit Conversion Tail Initialization/tail processing/tail initialization ==
  tail : Inport
  Trigger : TriggerPort  PortDimensions=1
  tail_0 : Outport  InitialOutput=0
  wires:
  tail/1 -> tail_0/1

== system et_robocon_zack_stepup/State Estimation/Gyro Processing/Compute psi/Very Low Pass Filter ==
  In1 : Inport
  Gain2 : Gain  Gain=0.004
  Gain3 : Gain  Gain=0.996
  Sum2 : Sum  Inputs=|++
  Unit Delay External IC : simulink/Additional Math & Discrete/Additional Discrete/Unit Delay External IC  tsamp=-1
  Out1 : Outport
  wires:
  Gain3/1 -> Sum2/2
  Sum2/1 -> Out1/1, Unit Delay External IC/1
  Gain2/1 -> Sum2/1
  Unit Delay External IC/1 -> Gain3/1
  In1/1 -> Gain2/1, Unit Delay External IC/2

== system et_robocon_zack_stepup/State Estimation/StateEstimation/Process theta1/Enabled Subsystem ==
  x : Inport
  Enable : EnablePort
  x0 : Outport  InitialOutput=0
  wires:
  x/1 -> x0/1

== system et_robocon_zack_stepup/State Estimation/StateEstimation/Process theta1/LPF and deriv ==
  theta : Inport
  Gain : Gain  Gain=1/0.004
  Low Pass Filter : DiscreteFilter  Numerator=[.2]  Denominator=[1 -0.8]
  Sum3 : Sum  Inputs=+-
  Unit Delay : UnitDelay  SampleTime=-1
  theta_dot : Outport
  wires:
  Unit Delay/1 -> Sum3/2
  Gain/1 -> Unit Delay/1, Sum3/1
  Sum3/1 -> theta_dot/1  "theta_dot"
  Low Pass Filter/1 -> Gain/1
  theta/1 -> Low Pass Filter/1

== system et_robocon_zack_stepup/State Estimation/StateEstimation/Process theta1/LPF and deriv1 ==
  theta_dot : Inport
  Gain : Gain  Gain=1/0.004
  Low Pass Filter : DiscreteFilter  Numerator=[.2]  Denominator=[1 -0.8]
  Sum3 : Sum  Inputs=+-
  Unit Delay : UnitDelay  SampleTime=-1
  theta_dot_dot : Outport
  wires:
  theta_dot/1 -> Low Pass Filter/1
  Low Pass Filter/1 -> Gain/1
  Sum3/1 -> theta_dot_dot/1  "theta_dot_dot"
  Gain/1 -> Sum3/1, Unit Delay/1
  Unit Delay/1 -> Sum3/2

== system et_robocon_zack_stepup/State Estimation/StateEstimation/Process theta1/Store x0 ==
  x : Inport
  Enable : EnablePort
  x0 : Outport  InitialOutput=0
  wires:
  x/1 -> x0/1

== stateflow chart et_robocon_zack_stepup/State Estimation/Gyro Processing/Reset Subsystem ==
  state CheckForReset
    bind: doProcess;
    entry: doProcess;
    during: doProcess;
  (default) -> CheckForReset
  CheckForReset -> CheckForReset : [init_flag == 1]
  data: init_flag input
  events: doProcess output FUNCTION_CALL_EVENT

== stateflow chart et_robocon_zack_stepup/Main Controller ==
  state restore
  state emergency_stop
    entry:
    debugFlag = uint16(9999);
  state normal_operation_modes
    state gyro_calibration_mode
    state light_sensor_calibration_mode
    state line_tracking_mode
    state see_saw_mode
    state limbo_mode
    state parking_mode
    state WeShouldNotBeHere
    (default) -> (junction 12) : {
        | current_mode_status = OperationModeStatusEnum.IN_PROGRESS;
        | }
    (junction 12) -> gyro_calibration_mode [order 1] : [  current_mode == OperationModeEnum.GYRO_CALIBRATION ]
    (junction 12) -> (junction 13) [order 2]
    (junction 13) -> light_sensor_calibration_mode [order 1] : [ current_mode == OperationModeEnum.LIGHT_SENSOR_CALIBRATION ]
    (junction 13) -> (junction 14) [order 2]
    (junction 14) -> line_tracking_mode [order 1] : [ current_mode == OperationModeEnum.LINE_TRACKING ]
    (junction 14) -> (junction 15) [order 2]
    (junction 15) -> see_saw_mode [order 1] : [ current_mode == OperationModeEnum.SEE_SAW ]
    (junction 15) -> (junction 17) [order 2]
    (junction 17) -> limbo_mode [order 1] : [  current_mode == OperationModeEnum.LIMBO ]
    (junction 17) -> (junction 19) [order 2]
    (junction 19) -> parking_mode [order 1] : [  current_mode == OperationModeEnum.PARKING ]
    (junction 19) -> (junction 99) [order 2]
    (junction 99) -> WeShouldNotBeHere
  (default) -> (junction 38) : {initFlags = Init_Bus0;}
  (junction 37) -> (junction 38)
  (junction 43) -> (junction 37)
  (junction 38) -> (junction 39) : { current_mode_index = uint8( 0 ); }
  (junction 40) -> (junction 39)
  restore -> (junction 40) : [ false == touch ]
  (junction 39) -> (junction 41) : {current_mode_status = OperationModeStatusEnum.NOT_STARTED;}
  normal_operation_modes -> (junction 40) [order 2] : [ current_mode_status == OperationModeStatusEnum.SUCCESSFULLY_COMPLETED ]
  (junction 42) -> (junction 41)
  (junction 41) -> (junction 44) : { current_mode_index = current_mode_index + uint8( 1 ); }
  (junction 47) -> (junction 42)
  emergency_stop -> restore : [ true == touch ]
  (junction 44) -> (junction 43) [order 1] : [ numel( TRACK_MODE_LIST ) < current_mode_index ]
      | % If the "current_mode_index" has exceeded the number
      | % of elements in the list, it should "wrap" back to the start.
  (junction 44) -> (junction 45) [order 2]
  (junction 45) -> (junction 46) : {current_mode = TRACK_MODE_LIST( current_mode_index );}
  (junction 46) -> (junction 47) [order 1] : [  current_mode == OperationModeEnum.SKIP ]
  (junction 46) -> normal_operation_modes [order 2]
  normal_operation_modes -> emergency_stop [order 1] : [ true == fall_detection_input ]
      | {current_mode_status = OperationModeStatusEnum.ABORTED;}
  data: PWM output Bus: PWM_bus size=1; TRACK_MODE_LIST parameter Enum: OperationModeEnum; current_mode_index local uint8; current_mode data_store_memory; states input Bus: States_Bus size=1; fall_detection_input input; current_mode_status data_store_memory; sensors input Bus: Sensors_Bus size=1; lightCalib data_store_memory; debugFlag output uint16 size=1; BT_status_out output single size=1; touch input single size=1; initFlags output Bus: Init_Bus size=1; Init_Bus0 parameter Bus: Init_Bus size=1; balancerStates_Bus0 parameter Bus: Balancer_States_Bus size=1

== stateflow chart et_robocon_zack_stepup/State Estimation/StateEstimation/Reset Subsystem ==
  state CheckForReset
    bind: doProcess;
    entry: doProcess;
    during: doProcess;
  (default) -> CheckForReset
  CheckForReset -> CheckForReset : [init_flag == 1]
  data: init_flag input
  events: doProcess output FUNCTION_CALL_EVENT
